simulink model "image_process"  (R2018b)
settings: Solver=VariableStepAuto  StartTime=0.0  StopTime=10.0  RelTol=1e-3
libraries: visionanalysis x6, dspvision x4
settings Model: Creator=ysl  LastModifiedBy=ysl

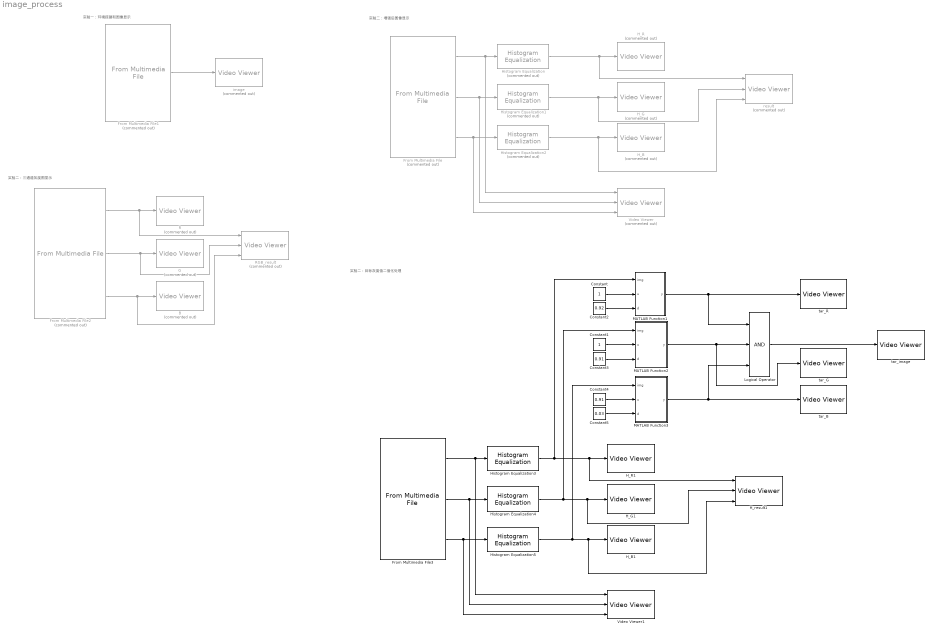
== system image_process ==
  note: 实验二：目标灰度值二值化处理
  note: 实验二：增强后图像显示
  note: 实验二：三通道灰度图显示
  note: 实验一：环境搭建和图像显示
  B : VideoViewer  Commented=on  FigPos=[7 482.666666666667 418 304]
  Constant : Constant
  Constant1 : Constant
  Constant2 : Constant  Value=0.92
  Constant3 : Constant  Value=0.91
  Constant4 : Constant  Value=0.91
  Constant5 : Constant  Value=0.03
  From Multimedia File : dspvision/From Multimedia File  Commented=on  inputFilename=D:\BaiduSyncdisk\000IFR\2022Balance\model\Task_vision\R-C.jpg  loop=on  numPlays=inf  outputStreams=Video only  videoDataType=single  audioDataType=int16  inheritSampleTime=on  userDefinedSampleTime=1/30  noAudioOutput=off  isIntensityVideo=off  fourcc=RGB  colorVideoFormat=Separate color signals  outputEOF=off  dataOrg=Column-major  audioFrameSize=1024  computeAudioFrameSize=off  outSamplingMode=Sample based
      settings: SourceProductBaseCode=VP
  From Multimedia File1 : dspvision/From Multimedia File  Commented=on  inputFilename=D:\BaiduSyncdisk\000IFR\2022Balance\model\Task_vision\R-C.jpg  loop=on  numPlays=inf  outputStreams=Video only  videoDataType=single  audioDataType=int16  inheritSampleTime=on  userDefinedSampleTime=1/30  noAudioOutput=off  isIntensityVideo=off  fourcc=RGB  colorVideoFormat=One multidimensional signal  outputEOF=off  dataOrg=Column-major  audioFrameSize=1024  computeAudioFrameSize=off  outSamplingMode=Sample based
      settings: SourceProductBaseCode=VP
  From Multimedia File2 : dspvision/From Multimedia File  Commented=on  inputFilename=D:\BaiduSyncdisk\000IFR\2022Balance\model\Task_vision\R-C.jpg  loop=on  numPlays=inf  outputStreams=Video only  videoDataType=single  audioDataType=int16  inheritSampleTime=on  userDefinedSampleTime=1/30  noAudioOutput=off  isIntensityVideo=off  fourcc=RGB  colorVideoFormat=Separate color signals  outputEOF=off  dataOrg=Column-major  audioFrameSize=1024  computeAudioFrameSize=off  outSamplingMode=Sample based
      settings: SourceProductBaseCode=VP
  From Multimedia File3 : dspvision/From Multimedia File  inputFilename=D:\BaiduSyncdisk\000IFR\2022Balance\model\Task_vision\R-C.jpg  loop=on  numPlays=inf  outputStreams=Video only  videoDataType=single  audioDataType=int16  inheritSampleTime=on  userDefinedSampleTime=1/30  noAudioOutput=off  isIntensityVideo=off  fourcc=RGB  colorVideoFormat=Separate color signals  outputEOF=off  dataOrg=Column-major  audioFrameSize=1024  computeAudioFrameSize=off  outSamplingMode=Sample based
      settings: SourceProductBaseCode=VP
  G : VideoViewer  Commented=on  FigPos=[359 490 418 304]
  H_B : VideoViewer  Commented=on  FigPos=[-197.666666666667 733.333333333333 1280 370]
  H_B1 : VideoViewer  FigPos=[-358.333333333333 793.333333333333 1280 583.333333333333]
  H_G : VideoViewer  Commented=on  FigPos=[-37 428 418 304]
  H_G1 : VideoViewer  FigPos=[-464.333333333333 807.333333333333 1280 583.333333333333]
  H_R : VideoViewer  Commented=on  FigPos=[421 426 418 304]
  H_R1 : VideoViewer  FigPos=[-283 760 1280 583.333333333333]
  H_result1 : VideoViewer  imagePorts=separate color signals  FigPos=[-333 793.333333333333 1280 583.333333333333]
  Histogram Equalization : visionanalysis/Histogram Equalization  Commented=on  specify=Uniform  numbins=64  src=Specify via dialog  hist=ones(1,64)
      settings: SourceProductName=Computer Vision System Toolbox  SourceProductBaseCode=VP
  Histogram Equalization1 : visionanalysis/Histogram Equalization  Commented=on  specify=Uniform  numbins=64  src=Specify via dialog  hist=ones(1,64)
      settings: SourceProductName=Computer Vision System Toolbox  SourceProductBaseCode=VP
  Histogram Equalization2 : visionanalysis/Histogram Equalization  Commented=on  specify=Uniform  numbins=64  src=Specify via dialog  hist=ones(1,64)
      settings: SourceProductName=Computer Vision System Toolbox  SourceProductBaseCode=VP
  Histogram Equalization3 : visionanalysis/Histogram Equalization  specify=Uniform  numbins=64  src=Specify via dialog  hist=ones(1,64)
      settings: SourceProductName=Computer Vision System Toolbox  SourceProductBaseCode=VP
  Histogram Equalization4 : visionanalysis/Histogram Equalization  specify=Uniform  numbins=64  src=Specify via dialog  hist=ones(1,64)
      settings: SourceProductName=Computer Vision System Toolbox  SourceProductBaseCode=VP
  Histogram Equalization5 : visionanalysis/Histogram Equalization  specify=Uniform  numbins=64  src=Specify via dialog  hist=ones(1,64)
      settings: SourceProductName=Computer Vision System Toolbox  SourceProductBaseCode=VP
  Logical Operator : Logic  Inputs=3  AllPortsSameDT=off  OutDataTypeStr=boolean
  MATLAB Function1 : MATLAB Function  TreatAsAtomicUnit=on
  MATLAB Function2 : MATLAB Function  TreatAsAtomicUnit=on
  MATLAB Function3 : MATLAB Function  TreatAsAtomicUnit=on
  R : VideoViewer  Commented=on  FigPos=[427.666666666667 481.333333333333 418 304]
  RGB_result : VideoViewer  Commented=on  imagePorts=separate color signals  FigPos=[-429 755.333333333333 1280 583.333333333333]
  Video Viewer : VideoViewer  Commented=on  imagePorts=separate color signals  FigPos=[-82.3333333333333 714 693.333333333333 440]
  Video Viewer1 : VideoViewer  imagePorts=separate color signals  FigPos=[24.3333333333333 664 693.333333333333 440]
  image : VideoViewer  Commented=on  FigPos=[320.333333333333 479.333333333333 418 304]
  result : VideoViewer  Commented=on  imagePorts=separate color signals  FigPos=[377.666666666667 587.333333333333 418 304]
  tar_B : VideoViewer  FigPos=[-215 790 1280 583.333333333333]
  tar_G : VideoViewer  FigPos=[-255.666666666667 798 1280 583.333333333333]
  tar_R : VideoViewer  FigPos=[-222.333333333333 905.333333333333 1280 583.333333333333]
  "tar_image " : VideoViewer  FigPos=[-239 737.333333333333 1280 583.333333333333]
  wires:
  From Multimedia File/1 -> Video Viewer/1, Histogram Equalization/1
  Histogram Equalization/1 -> result/1, H_R/1
  From Multimedia File/2 -> Video Viewer/2, Histogram Equalization1/1
  Histogram Equalization1/1 -> result/2, H_G/1
  From Multimedia File/3 -> Video Viewer/3, Histogram Equalization2/1
  Histogram Equalization2/1 -> result/3, H_B/1
  From Multimedia File1/1 -> image/1
  From Multimedia File2/1 -> RGB_result/1, R/1
  From Multimedia File2/2 -> RGB_result/2, G/1
  From Multimedia File2/3 -> RGB_result/3, B/1
  Histogram Equalization5/1 -> MATLAB Function3/1(img), H_result1/3, H_B1/1
  From Multimedia File3/2 -> Video Viewer1/2, Histogram Equalization4/1
  Histogram Equalization4/1 -> MATLAB Function2/1(img), H_result1/2, H_G1/1
  Histogram Equalization3/1 -> MATLAB Function1/1(img), H_result1/1, H_R1/1
  From Multimedia File3/1 -> Video Viewer1/1, Histogram Equalization3/1
  From Multimedia File3/3 -> Video Viewer1/3, Histogram Equalization5/1
  Constant/1 -> MATLAB Function1/2(u)
  Constant1/1 -> MATLAB Function2/2(u)
  Constant2/1 -> MATLAB Function1/3(d)
  Constant3/1 -> MATLAB Function2/3(d)
  Constant4/1 -> MATLAB Function3/2(u)
  Constant5/1 -> MATLAB Function3/3(d)
  MATLAB Function2/1(y) -> tar_G/1, Logical Operator/2
  MATLAB Function1/1(y) -> Logical Operator/1, tar_R/1
  MATLAB Function3/1(y) -> Logical Operator/3, tar_B/1
  Logical Operator/1 -> "tar_image "/1

== matlab function image_process/MATLAB Function1 ==
  data: img input; u input; y output; d input
function y = fcn(img,u,d)
[n,m] = size(img);
A = zeros(n,m);
for a = 1:n
    for b = 1:m
        if img(a,b) >= d && img(a,b) <= u
            A(a,b) = 1;
        else
            A(a,b) = 0;
        end
    end
end
y = A;

== matlab function image_process/MATLAB Function2 ==
  data: img input; u input; y output; d input
function y = fcn(img,u,d)
[n,m] = size(img);
A = zeros(n,m);
for a = 1:n
    for b = 1:m
        if img(a,b) >= d && img(a,b) <= u
            A(a,b) = 1;
        else
            A(a,b) = 0;
        end
    end
end
y = A;

== matlab function image_process/MATLAB Function3 ==
  data: img input; u input; y output; d input
function y = fcn(img,u,d)
[n,m] = size(img);
A = zeros(n,m);
for a = 1:n
    for b = 1:m
        if img(a,b) >= d && img(a,b) <= u
            A(a,b) = 1;
        else
            A(a,b) = 0;
        end
    end
end
y = A;
